simulink model "CoDIT_static"  (Simulink 8.5)
settings: Solver=ode45  StartTime=0.0  StopTime=30.0  RelTol=1e-3
values from neighbouring files (symbols this model uses):
  A = [0 1;-1 0]    [Consensus_algo.m]
  Ad = [0 1 1 0 0;1 0 0 0 0;1 0 0 -1 0;0 0 -1 0 1;0 0 0 1 0]    [Consensus_algo.m]
  B = [0;1]    [Consensus_algo.m]
  beta = 1.5    [Consensus_algo.m]
  C = [1 0;0 1]    [Consensus_algo.m]
  c2 = 1.2    [Consensus_algo.m]
  D = [0;0]    [Consensus_algo.m]
  Dp = [0 0 0 0 0;0 2 0 0 0;0 0 0 0 0;0 0 0 2 0;0 0 0 0 0]    [Consensus_algo.m]
  Fgain = -B'*P    [Consensus_algo.m]
  tau = 1    [Consensus_algo.m]    (also in mas.m = 1/lambda_2)
  x00 = [-2;6]    [Consensus_algo.m]
  x10 = [1;-4]    [Consensus_algo.m]
  x20 = [-4;-2]    [Consensus_algo.m]
  x30 = [3;8]    [Consensus_algo.m]
  x40 = [-5;-5]    [Consensus_algo.m]
  x50 = [2;-7]    [Consensus_algo.m]
settings Model: Creator=User  LastModifiedBy=User
settings DataIOCC: SignalLoggingSaveFormat=Dataset
settings OptimizationCC: ExpressionDepthLimit=128
settings DebuggingCC: UnderspecifiedInitializationDetection=Simplified  MergeDetectMultiDrivingBlocksExec=error  FcnCallInpInsideContextMsg=EnableAllAsError  StateNameClashWarn=none
settings GRTTargetCC: CombineOutputUpdateFcns=on  GRTInterface=off

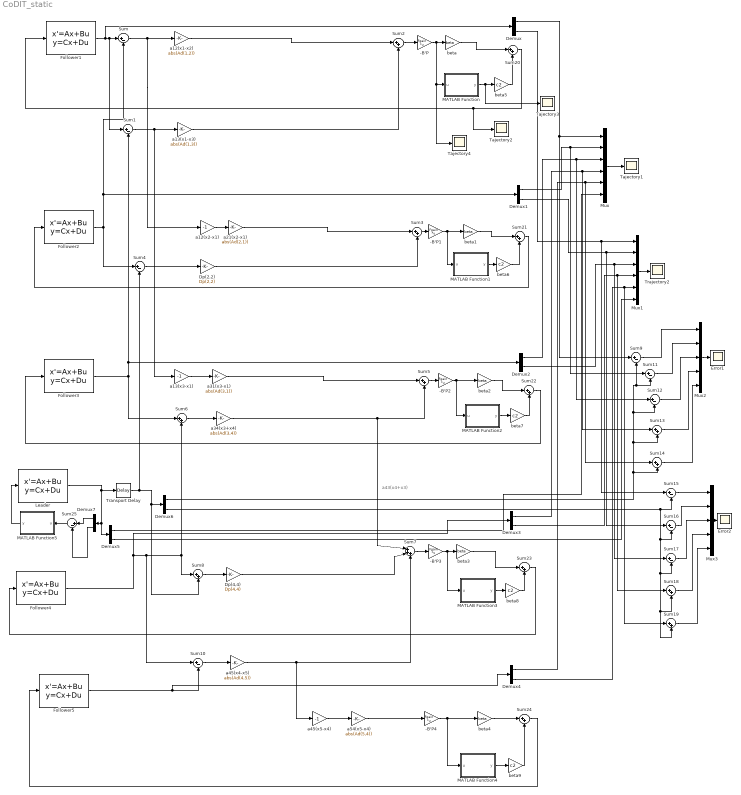
== system CoDIT_static ==
  note: a43(x4+x3)
  -B'P{,1..4} (5 alike) : Gain  Gain=Fgain  Multiplication=Matrix(K*u)
  Demux{,1..7} (8 alike) : Demux  Outputs=2
  Dp(2,2) : Gain  Gain=Dp(2,2)
  Dp(4,4) : Gain  Gain=Dp(4,4)
  Error1 : Scope
      settings: SaveName=e1
  Error2 : Scope
      settings: SaveName=e2
  Follower1 : StateSpace  A=A  B=B  C=C  D=D  X0=x10
  Follower2 : StateSpace  A=A  B=B  C=C  D=D  X0=x20
  Follower3 : StateSpace  A=A  B=B  C=C  D=D  X0=x30
  Follower4 : StateSpace  A=A  B=B  C=C  D=D  X0=x40
  Follower5 : StateSpace  A=A  B=B  C=C  D=D  X0=x50
  Leader : StateSpace  A=A  B=B  C=C  D=D  X0=x00
  MATLAB Function : MATLAB Function  TreatAsAtomicUnit=on
  MATLAB Function1 : MATLAB Function  TreatAsAtomicUnit=on
  MATLAB Function2 : MATLAB Function  TreatAsAtomicUnit=on
  MATLAB Function3 : MATLAB Function  TreatAsAtomicUnit=on
  MATLAB Function4 : MATLAB Function  TreatAsAtomicUnit=on
  MATLAB Function5 : MATLAB Function  TreatAsAtomicUnit=on
  Mux : Mux  Inputs=6
  Mux1 : Mux  Inputs=6
  Mux2 : Mux  Inputs=5
  Mux3 : Mux  Inputs=5
  Sum{,1,4,9..12,15..17,25} (11 alike) : Sum  Inputs=|+-
  Sum{2..3,5..6,8,13..14,18..24} (14 alike) : Sum  Inputs=|++
  Sum7 : Sum  Inputs=|+++
  Tajectory{1..4} (4 alike) : Scope
      Tajectory1 settings: SaveName=trajx1
      Tajectory2 settings: SaveName=trajx
      Tajectory3 settings: SaveName=trajx3
      Tajectory4 settings: SaveName=trajx4
  Trajectory2 : Scope
      settings: SaveName=trajx2
  Transport Delay : TransportDelay  DelayTime=tau  InitialOutput=[0;0]
  a12(x1-x2) : Gain  Gain=abs(Ad(1,2))
  a12(x2-x1) : Gain  Gain=-1
  a13(x1-x3) : Gain  Gain=abs(Ad(1,3))
  a13(x3-x1) : Gain  Gain=-1
  a21(x2-x1) : Gain  Gain=abs(Ad(2,1))
  a31(x3-x1) : Gain  Gain=abs(Ad(3,1))
  a34(x3+x4) : Gain  Gain=abs(Ad(3,4))
  a45(x4-x5) : Gain  Gain=abs(Ad(4,5))
  a45(x5-x4) : Gain  Gain=-1
  a54(x5-x4) : Gain  Gain=abs(Ad(5,4))
  beta{,1..4} (5 alike) : Gain  Gain=beta
  beta{5..9} (5 alike) : Gain  Gain=c2
  wires:
  Follower1/1 -> Demux/1, Sum1/1, Sum/1
  Follower2/1 -> Demux1/1, Sum/2, Sum4/1
  Sum/1 -> a12(x2-x1)/1, a12(x1-x2)/1
  Follower3/1 -> Demux2/1, Sum1/2, Sum6/1
  Sum1/1 -> a13(x3-x1)/1, a13(x1-x3)/1
  a13(x1-x3)/1 -> Sum2/2
  a12(x1-x2)/1 -> Sum2/1
  a12(x2-x1)/1 -> a21(x2-x1)/1
  Sum2/1 -> -B'P/1
  a21(x2-x1)/1 -> Sum3/1
  Sum3/1 -> -B'P1/1
  -B'P1/1 -> MATLAB Function1/1(u), beta1/1
  Sum4/1 -> Dp(2,2)/1
  Dp(2,2)/1 -> Sum3/2
  a13(x3-x1)/1 -> a31(x3-x1)/1
  a31(x3-x1)/1 -> Sum5/1
  Follower4/1 -> Demux3/1, Sum10/1, Sum8/1, Sum6/2
  Sum6/1 -> a34(x3+x4)/1
  a34(x3+x4)/1 -> Sum7/1, Sum5/2
  Sum5/1 -> -B'P2/1
  -B'P2/1 -> MATLAB Function2/1(u), beta2/1
  Dp(4,4)/1 -> Sum7/2
  Sum8/1 -> Dp(4,4)/1
  Sum7/1 -> -B'P3/1
  -B'P3/1 -> MATLAB Function3/1(u), beta3/1
  Follower5/1 -> Demux4/1, Sum10/2
  Sum10/1 -> a45(x4-x5)/1
  a45(x4-x5)/1 -> Sum7/3, a45(x5-x4)/1
  a45(x5-x4)/1 -> a54(x5-x4)/1
  a54(x5-x4)/1 -> -B'P4/1
  -B'P4/1 -> MATLAB Function4/1(u), beta4/1
  Leader/1 -> Transport Delay/1, Demux5/1, Demux7/1
  Demux/1 -> Sum9/1, Mux/1
  Demux1/1 -> Sum11/1, Mux/2
  Demux2/1 -> Sum12/1, Mux/3
  Demux3/1 -> Sum13/1, Mux/4
  Demux4/1 -> Sum14/1, Mux/5
  Demux5/1 -> Mux/6
  Mux/1 -> Tajectory1/1
  Demux/2 -> Sum15/1, Mux1/1
  Demux1/2 -> Sum16/1, Mux1/2
  Demux2/2 -> Sum17/1, Mux1/3
  Demux3/2 -> Sum18/1, Mux1/4
  Demux4/2 -> Sum19/1, Mux1/5
  Demux5/2 -> Mux1/6
  Mux1/1 -> Trajectory2/1
  Demux6/1 -> Sum14/2, Sum13/2, Sum12/2, Sum11/2, Sum9/2
  Sum9/1 -> Mux2/1
  Mux2/1 -> Error1/1
  Sum11/1 -> Mux2/2
  Sum12/1 -> Mux2/3
  Sum13/1 -> Mux2/4
  Sum14/1 -> Mux2/5
  Mux3/1 -> Error2/1
  Sum15/1 -> Mux3/1
  Demux6/2 -> Sum18/2, Sum19/2, Sum17/2, Sum16/2, Sum15/2
  Sum16/1 -> Mux3/2
  Sum17/1 -> Mux3/3
  Sum18/1 -> Mux3/4
  Sum19/1 -> Mux3/5
  -B'P/1 -> Tajectory4/1, MATLAB Function/1(u), beta/1
  MATLAB Function/1(y) -> Tajectory3/1, beta5/1
  beta/1 -> Sum20/1
  beta5/1 -> Sum20/2
  Sum20/1 -> Tajectory2/1, Follower1/1
  beta1/1 -> Sum21/1
  MATLAB Function1/1(y) -> beta6/1
  beta6/1 -> Sum21/2
  Sum21/1 -> Follower2/1
  beta7/1 -> Sum22/2
  beta2/1 -> Sum22/1
  MATLAB Function2/1(y) -> beta7/1
  Sum22/1 -> Follower3/1
  beta3/1 -> Sum23/1
  MATLAB Function3/1(y) -> beta8/1
  beta8/1 -> Sum23/2
  Sum23/1 -> Follower4/1
  MATLAB Function4/1(y) -> beta9/1
  beta4/1 -> Sum24/1
  beta9/1 -> Sum24/2
  Sum24/1 -> Follower5/1
  Transport Delay/1 -> Sum8/2, Demux6/1, Sum4/2
  Sum25/1 -> MATLAB Function5/1(u)
  Demux7/1 -> Sum25/1
  Demux7/2 -> Sum25/2
  MATLAB Function5/1(y) -> Leader/1

== matlab function MATLAB Function1 ==
  data: u input double; y output double
function y = fcn(u)
%#codegen

y = sign(u);

== matlab function MATLAB Function ==
  data: u input double; y output double
function y = fcn(u)
%#codegen

y = sign(u);

== matlab function MATLAB Function2 ==
  data: u input double; y output double
function y = fcn(u)
%#codegen

y = sign(u);

== matlab function MATLAB Function3 ==
  data: u input double; y output double
function y = fcn(u)
%#codegen

y = sign(u);

== matlab function MATLAB Function4 ==
  data: u input double; y output double
function y = fcn(u)
%#codegen

y = sign(u);

== matlab function MATLAB Function5 ==
  data: u input double; y output double
function y = fcn(u)
%#codegen

y = sin(u);
